simulink model "Diode_Rectifier_Six_Phase_Rload"  (R2018b)
settings: Solver=VariableStepAuto  StartTime=0.0  StopTime=0.04  RelTol=1e-3
libraries: powerlib x24
settings Model: Creator=A.hey  LastModifiedBy=A.hey

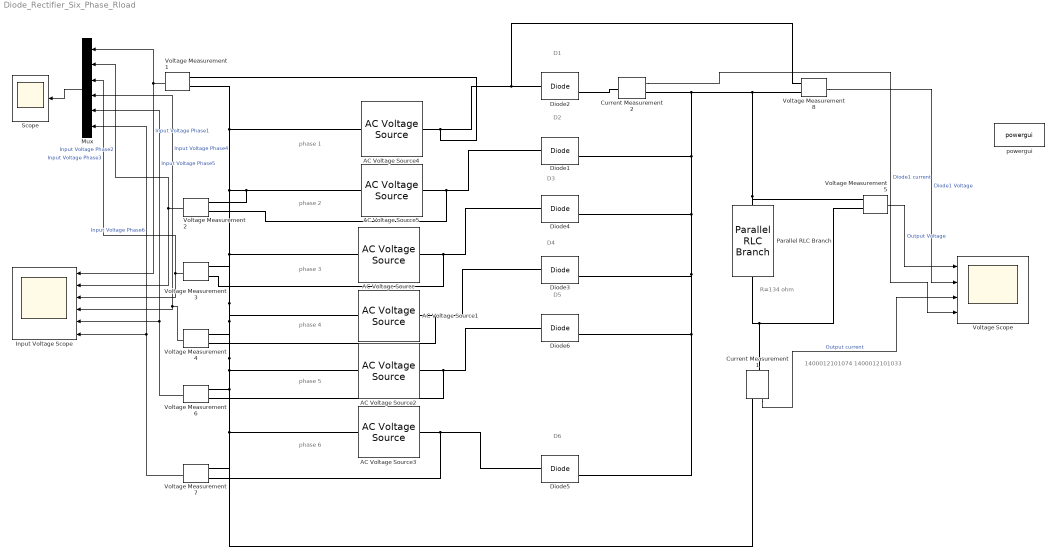
== system Diode_Rectifier_Six_Phase_Rload ==
  note: D1
  note: D2
  note: D4
  note: D3
  note: D6
  note: D5
  note: R=134 ohm
  note: 1400012101074
      | 1400012101033
  note: phase 1
  note: phase 3
  note: phase 2
  note: phase 4
  note: phase 5
  note: phase 6
  AC Voltage Source : powerlib/Electrical Sources/AC Voltage Source  Amplitude=220  Phase=-180  Frequency=50  SampleTime=0  Measurements=None  BusType=swing  Pref=10e3  Qref=0  Qmin=-inf  Qmax=+inf
  AC Voltage Source1 : powerlib/Electrical Sources/AC Voltage Source  Amplitude=220  Phase=-240  Frequency=50  SampleTime=0  Measurements=None  BusType=swing  Pref=10e3  Qref=0  Qmin=-inf  Qmax=+inf
  AC Voltage Source2 : powerlib/Electrical Sources/AC Voltage Source  Amplitude=220  Phase=-300  Frequency=50  SampleTime=0  Measurements=None  BusType=swing  Pref=10e3  Qref=0  Qmin=-inf  Qmax=+inf
  AC Voltage Source3 : powerlib/Electrical Sources/AC Voltage Source  Amplitude=220  Phase=-360  Frequency=50  SampleTime=0  Measurements=None  BusType=swing  Pref=10e3  Qref=0  Qmin=-inf  Qmax=+inf
  AC Voltage Source4 : powerlib/Electrical Sources/AC Voltage Source  Amplitude=220  Phase=-60  Frequency=50  SampleTime=0  Measurements=None  BusType=swing  Pref=10e3  Qref=0  Qmin=-inf  Qmax=+inf
  AC Voltage Source5 : powerlib/Electrical Sources/AC Voltage Source  Amplitude=220  Phase=-120  Frequency=50  SampleTime=0  Measurements=None  BusType=swing  Pref=10e3  Qref=0  Qmin=-inf  Qmax=+inf
  Current Measurement1 : powerlib/Measurements/Current Measurement  PhasorSimulation=off  OutputType=Complex  PSBequivalent=0
  Current Measurement2 : powerlib/Measurements/Current Measurement  PhasorSimulation=off  OutputType=Complex  PSBequivalent=0
  Diode{1..6} (6 alike) : powerlib/Power Electronics/Diode  Ron=0.001  Lon=0  Vf=0.8  IC=0  UseSnubber=0  Rs=500  Cs=250e-9  Measurements=on
  "Input Voltage Scope " : Scope  NumInputPorts=6
  Mux : Mux  Inputs=6
  Parallel RLC Branch : powerlib/Elements/Parallel RLC Branch  LConnTagsString=a  RConnTagsString=__new0  BranchType=R  Resistance=134  Inductance=1e-3  SetiL0=off  InitialCurrent=0  Capacitance=1e-6  Setx0=off  InitialVoltage=0  Measurements=None
  Scope : Scope
  Voltage Measurement{1..8} (8 alike) : powerlib/Measurements/Voltage Measurement  PhasorSimulation=off  OutputType=Complex  PSBequivalent=0
  "Voltage Scope " : Scope  NumInputPorts=4
  powergui : powerlib/powergui  Priority=1  SimulationMode=Continuous  SampleTime=50e-6  frequency=60  Iterations=50  frequencyindice=50  Pbase=100e6  ErrMax=1e-4  UnitsV=kV  UnitsW=MW  buscounter=0  FunctionMessages=off  echomessages=off  EnableUseOfTLC=off  CurrentSourceSwitches=off  DisableSnubberDevices=off  DisableRonSwitches=off  DisableVfSwitches=off  DisplayEquations=off  SolverType=Tustin/Backward Euler (TBE)  Interpol=off  ExternalGateDelay=off  methode=off  Ts=100  x0status=blocks  SPID=on  SwTol=0  HookPort=off  RestoreLinks=warning  ResistiveCurrentMeasurement=off  Frange=[0:2:500]  Ylog=off  Xlog=on  ShowGrid=off  save=off  variable=ZData  structure=0  ZoomFFT=off  StartTime=0.0  cycles=1  DisplayStyle=1  fundamental=60  FreqAxis=off  MaxFrequency=1000  frequencyindicesteady=1  RmsSteady=1  display=off
  wires:
  Voltage Measurement5/1 -> "Voltage Scope "/1  "Output Voltage"
  Voltage Measurement1/1 -> Mux/1, "Input Voltage Scope "/1  "Input Voltage Phase1"
  Voltage Measurement2/1 -> Mux/2, "Input Voltage Scope "/2  "Input Voltage Phase2"
  Voltage Measurement3/1 -> Mux/3, "Input Voltage Scope "/3  "Input Voltage Phase3"
  Voltage Measurement4/1 -> Mux/4, "Input Voltage Scope "/4  "Input Voltage Phase4"
  Voltage Measurement6/1 -> Mux/5, "Input Voltage Scope "/5  "Input Voltage Phase5"
  Voltage Measurement7/1 -> Mux/6, "Input Voltage Scope "/6  "Input Voltage Phase6"
  Voltage Measurement8/1 -> "Voltage Scope "/2  "Diode1 Voltage"
  Current Measurement1/1 -> "Voltage Scope "/3  "Output current"
  Current Measurement2/1 -> "Voltage Scope "/4  "Diode1 current"
  Mux/1 -> Scope/1
  connections:
  Diode2/LConn1 -- Voltage Measurement8/LConn1 -- Voltage Measurement1/LConn1 -- AC Voltage Source4/RConn1
  AC Voltage Source5/RConn1 -- Voltage Measurement2/LConn1 -- Diode1/LConn1
  AC Voltage Source1/RConn1 -- Voltage Measurement4/LConn1 -- Diode3/LConn1
  AC Voltage Source/RConn1 -- Voltage Measurement3/LConn1 -- Diode4/LConn1
  AC Voltage Source3/RConn1 -- Voltage Measurement7/LConn1 -- Diode5/LConn1
  AC Voltage Source2/RConn1 -- Voltage Measurement6/LConn1 -- Diode6/LConn1
  Diode5/RConn1 -- Diode3/RConn1 -- Voltage Measurement8/LConn2 -- Voltage Measurement5/LConn1 -- Parallel RLC Branch/LConn1 -- Current Measurement2/RConn1 -- Diode1/RConn1 -- Diode4/RConn1 -- Diode6/RConn1
  AC Voltage Source4/LConn1 -- Voltage Measurement1/LConn2 -- Voltage Measurement2/LConn2 -- AC Voltage Source5/LConn1 -- Voltage Measurement3/LConn2 -- Voltage Measurement4/LConn2 -- Voltage Measurement6/LConn2 -- Current Measurement1/RConn1 -- Voltage Measurement7/LConn2 -- AC Voltage Source3/LConn1 -- AC Voltage Source2/LConn1 -- AC Voltage Source1/LConn1 -- AC Voltage Source/LConn1
  Voltage Measurement5/LConn2 -- Parallel RLC Branch/RConn1 -- Current Measurement1/LConn1
  Current Measurement2/LConn1 -- Diode2/RConn1
